simulink model "untitled2"  (R2020a)
settings: Solver=FixedStepAuto  StartTime=0.0  StopTime=inf  FixedStep=0.001  RelTol=1e-3
model workspace (MAT data in the model file):
  Kd = 1
  Ki = 10
  Kp = 1
  kd = 1
undefined symbols (not defined in the file): DiscIntNeverNeededParam
libraries: simulink x1
settings Model: Creator=Vulca  LastModifiedBy=Vulca
settings OptimizationCC: DefaultParameterBehavior=Inlined  EnhancedBackFolding=on  PassReuseOutputArgsAs=Individual arguments  ZeroExternalMemoryAtStartup=off  ZeroInternalMemoryAtStartup=off  OptimizeBlockOrder=speed  DifferentSizesBufferReuse=on  OptimizationCustomize=off  EfficientTunableParamExpr=on
settings DebuggingCC: ParameterTunabilityLossMsg=error
settings SFSimCC: MATLABDynamicMemAlloc=off
settings RTWCC: SystemTargetFile=ert.tlc  TemplateMakefile=ert_default_tmf  TargetLang=C++
settings CodeAppCC: ForceParamTrailComments=on  IgnoreCustomStorageClasses=off  OperatorAnnotations=on  SimulinkDataObjDesc=on  SFDataObjDesc=on  InsertBlockDesc=on
settings ERTTargetCC: TargetLangStandard=C++03 (ISO)  GenerateSampleERTMain=on  MultiInstanceERTCode=on  CodeInterfacePackaging=C++ class  InlinedParameterPlacement=NonHierarchical  RootIOFormat=Structure reference  ERTCustomFileTemplate=example_file_process.tlc

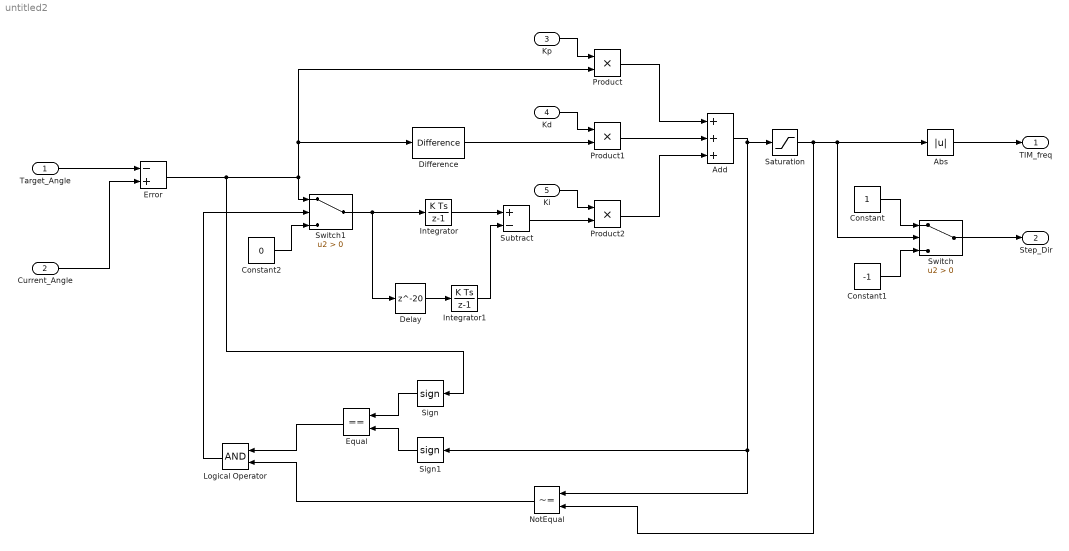
== system untitled2 ==
  Target_Angle : Inport
  Current_Angle : Inport  Port=2
  Kp : Inport  Port=3
  Kd : Inport  Port=4
  Ki : Inport  Port=5
  Abs : Abs
  Add : Sum  Inputs=+++
  Constant : Constant
  Constant1 : Constant  Value=-1
  Constant2 : Constant  Value=0
  Delay : Delay  DelayLength=20  InitialCondition=0
  Difference : simulink/Discrete/Difference  ICPrevInput=0.0  OutMin=[]  OutMax=[]  OutDataType=fixdt(1, 16)  OutScaling=2^-10  DoSatur=off
  Equal : RelationalOperator  Operator===  OutDataTypeStr=boolean  RndMeth=Simplest
  Error : Sum  Inputs=-+
  Integrator : DiscreteIntegrator  ICPrevOutput=DiscIntNeverNeededParam  ICPrevScaledInput=DiscIntNeverNeededParam  mask(DiscretizedDiscreteIntegrator){}
      mask init:
      | %zoh
  Integrator1 : DiscreteIntegrator  ICPrevOutput=DiscIntNeverNeededParam  ICPrevScaledInput=DiscIntNeverNeededParam  mask(DiscretizedDiscreteIntegrator){}
      mask init:
      | %zoh
  Logical Operator : Logic  AllPortsSameDT=off  OutDataTypeStr=boolean
  NotEqual : RelationalOperator  Operator=~=  OutDataTypeStr=boolean  RndMeth=Simplest
  Product : Product
  Product1 : Product
  Product2 : Product
  Saturation : Saturate  UpperLimit=2000  LowerLimit=-2000
  Sign : Signum
  Sign1 : Signum
  Subtract : Sum  Inputs=+-
  Switch : Switch  Criteria=u2 > Threshold
  Switch1 : Switch  Criteria=u2 > Threshold
  TIM_freq : Outport
  Step_Dir : Outport  Port=2
  wires:
  Target_Angle/1 -> Error/1
  Current_Angle/1 -> Error/2
  Integrator1/1 -> Subtract/2
  Error/1 -> Switch1/1, Difference/1, Product/2, Sign/1
  Integrator/1 -> Subtract/1
  Delay/1 -> Integrator1/1
  Product/1 -> Add/1
  Add/1 -> Saturation/1, NotEqual/1, Sign1/1
  Kp/1 -> Product/1
  Kd/1 -> Product1/1
  Difference/1 -> Product1/2
  Product1/1 -> Add/2
  Ki/1 -> Product2/1
  Subtract/1 -> Product2/2
  Product2/1 -> Add/3
  Saturation/1 -> NotEqual/2, Switch/2, Abs/1
  Constant/1 -> Switch/1
  Constant1/1 -> Switch/3
  Abs/1 -> TIM_freq/1
  Switch/1 -> Step_Dir/1
  Switch1/1 -> Delay/1, Integrator/1
  Logical Operator/1 -> Switch1/2
  Constant2/1 -> Switch1/3
  Sign/1 -> Equal/1
  Sign1/1 -> Equal/2
  Equal/1 -> Logical Operator/1
  NotEqual/1 -> Logical Operator/2
